simulink model "host_visualization"  (R2018b)
settings: Solver=FixedStepAuto  StartTime=0.0  StopTime=inf  FixedStep=0.002  RelTol=1e-3
model workspace (MAT data in the model file):
  P_Sim_LowPassVisualization = Simulink.Parameter
  P_Sim_LowPassVisualization.Value = 0.03
  P_Sim_LowPassVisualization.DataType = 'auto'
  P_Sim_LowPassVisualization.Dimensions = [1 1]
libraries: misc x6, sim3dlib x3, simulink x1, xpcrtudplib x1, xpcutilitieslib x1
settings Model: EnablePacing=on  Creator=speedgoat  LastModifiedBy=ge34qer

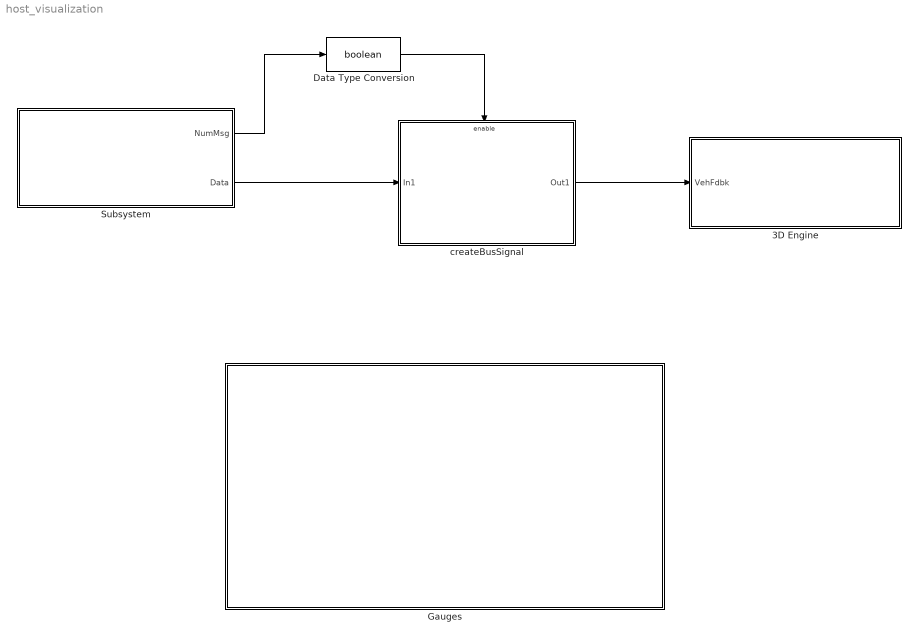
== system host_visualization ==
  3D Engine : Subsystem  VariantControlMode=Label  Variant=on  LabelModeActiveChoice=1  mask(3D Engine){engine3D=Enabled, SceneDesc=Straight road, dt3D=0.02}
      mask prompts: engine3D "3D Engine"; SceneDesc "Scene Description:"; dt3D "Engine frame rate, dt3D [s]:"
      mask help: This subsystem contains the interface blocks which permit the display of the vehicle in 3D virtual environment. Enable it to view the simulation progress, disable it to inhibit the display.
      mask init:
      | switch get_param(gcb,'engine3D')
      |     case 'Disabled'
      |         set_param(gcb,'OverrideUsingVariant','0')
      |         try
      |             set_param([bdroot '/Environment/Ground Feedback'],'OverrideUsingVariant','0')
      |         catch
      |             disp('No ground feedback sensor found')
      |         end
      |     case 'Enabled'
      |         set_param(gcb,'OverrideUsingVariant','1')
      |         try
      |             set_param([bdroot '/Environment/Ground Feedback'],'OverrideUsingVariant','1')
      |         catch
      |             disp('No ground feedback sensor found')
      |         end
      |     otherwise
      |         set_param(gcb,'OverrideUsingVariant','0')
      | end
      settings: AttributesFormatString=%<engine3D>
      mask Help: eval('vdynblkshelp(''vdynblksscenecameraray'')');
      mask TypeOptions engine3D: Enabled | Disabled
      mask Callback engine3D:
      | switch get_param(gcb,'engine3D')
      |     case 'Disabled'
      |         set_param(gcb,'OverrideUsingVariant','0')
      |     case 'Enabled'
      |        set_param(gcb,'OverrideUsingVariant','1')
      |     otherwise
      |        set_param(gcb,'OverrideUsingVariant','0')
      | end
      mask TypeOptions SceneDesc:
      | 3D Engine/Simulation 3D Engine
      | 1/SceneDesc
      mask Display: disp('3D Engine')
  Data Type Conversion : DataTypeConversion  OutDataTypeStr=boolean
  Gauges : Subsystem
  Subsystem : Subsystem
  createBusSignal : Subsystem
  wires:
  createBusSignal/1(Out1) -> 3D Engine/1(VehFdbk)
  Subsystem/1(NumMsg) -> Data Type Conversion/1
  Data Type Conversion/1 -> createBusSignal/Enable
  Subsystem/2(Data) -> createBusSignal/1(In1)

== system host_visualization/3D Engine ==
  note: 1) Add Subsystem or Model blocks as valid variant choices.
      | 2) You cannot connect blocks at this level. At simulation, connectivity is automatically
      | determined, based on the active variant and port name matching.
  VehFdbk : Inport
  3D Engine : Subsystem  VariantControl=1
  3D Engine Disabled : Subsystem  VariantControl=0

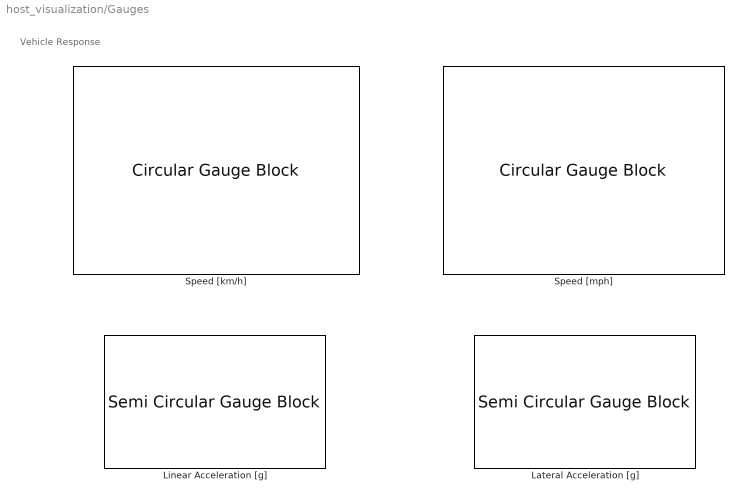
== system host_visualization/Gauges ==
  note: Vehicle Response
  Lateral Acceleration [g] : SemiCircularGaugeBlock  WebBlockId=331  LabelPosition=Hide  ScaleMin=-1.6000000000000001  ScaleMax=1.6000000000000001
  Linear Acceleration [g] : SemiCircularGaugeBlock  WebBlockId=343  LabelPosition=Hide  ScaleMin=-1.6000000000000001  ScaleMax=1.6000000000000001
  Speed [km/h] : CircularGaugeBlock  WebBlockId=332  LabelPosition=Hide  ScaleMax=210
  Speed [mph] : CircularGaugeBlock  WebBlockId=339  LabelPosition=Hide  ScaleMax=130

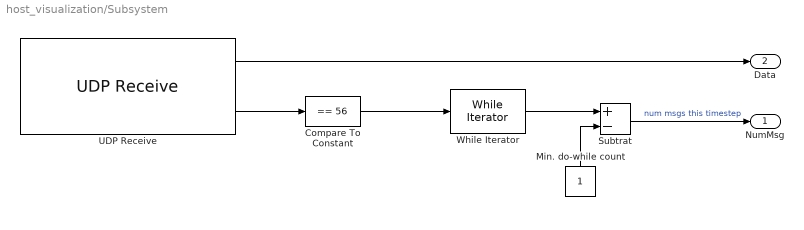
== system host_visualization/Subsystem ==
  Compare To Constant : simulink/Logic and Bit Operations/Compare To Constant  Priority=1  relop===  const=56  OutDataTypeStr=boolean
  Min. do-while count : Constant  OutDataTypeStr=int8  SampleTime=-1
  Subtrat : Sum  Inputs=+-
  UDP Receive : xpcrtudplib/UDP Receive  ipAddressVal=Use host-target connection  localPort=25000  rcvWidth=56  rcvFmAny=off  fmAddress=192.168.7.3  rcvMulticast=off  multicastAddress={}  maxUDPQueue=8  sampleTime=-1
      settings: SourceProductName=Simulink Real-Time
  While Iterator : WhileIterator  WhileBlockType=do-while  ShowIterationPort=on  OutputDataType=int16
  NumMsg : Outport
  Data : Outport  Port=2
  wires:
  Subtrat/1 -> NumMsg/1  "num msgs this timestep"
  Compare To Constant/1 -> While Iterator/1
  UDP Receive/1 -> Data/1
  Min. do-while count/1 -> Subtrat/2
  While Iterator/1 -> Subtrat/1
  UDP Receive/2 -> Compare To Constant/1

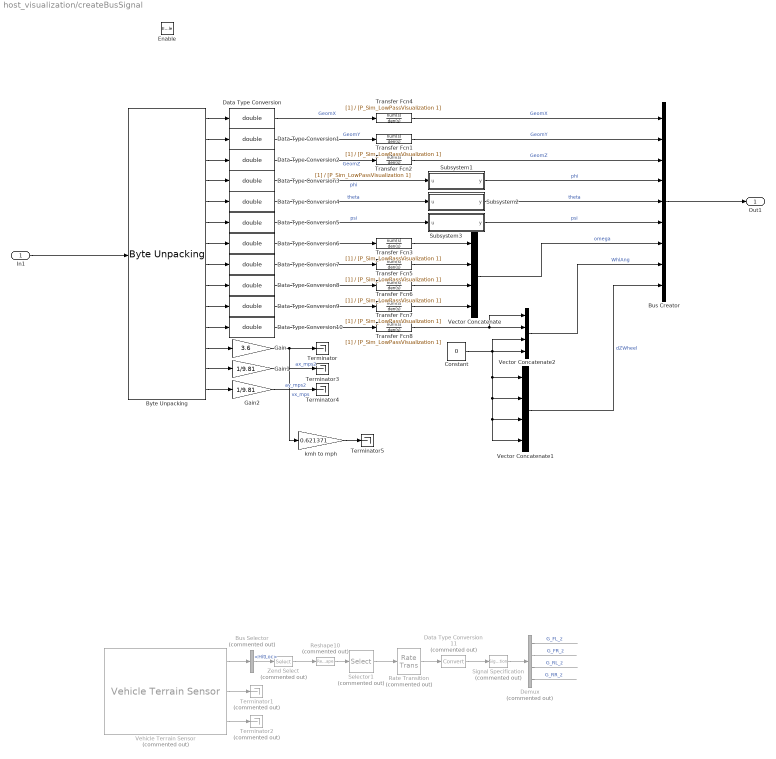
== system host_visualization/createBusSignal ==
  In1 : Inport
  Enable : EnablePort
  Bus Creator : BusCreator  Inputs=9
  Bus Selector : BusSelector  Commented=on  OutputSignals=HitLoc
  "Byte Unpacking " : xpcutilitieslib/Byte Unpacking   MaskUnpackedDataTypes={'single','single','single','single','single','single','single','single','single','single','single','single','single','single'}  MaskUnpackedDataSizes={[1],[1],[1],[1],[1],[1],[1],[1],[1],[1],[1],[1],[1],[1]}  MaskAlignment=1
      settings: SourceProductName=Simulink Real-Time  SourceProductBaseCode=XP
  Constant : Constant  Value=0  OutDataTypeStr=double  SampleTime=-1
  Data Type Conversion{,1..10} (11 alike) : DataTypeConversion  OutDataTypeStr=double
  Data Type Conversion11 : DataTypeConversion  Commented=on
  Demux : Demux  Commented=on
  Gain : Gain  Gain=3.6
  Gain1 : Gain  Gain=1/9.81
  Gain2 : Gain  Gain=1/9.81
  Rate Transition : RateTransition  Commented=on
  Reshape10 : Reshape  Commented=on  OutputDimensionality=Row vector (2-D)
  Selector1 : Selector  Commented=on  InputPortWidth=5  IndexOptions=Index vector (dialog)  Indices=[2:5]  OutputSizes=1
  Signal Specification : SignalSpecification  Commented=on  Unit=m
  Subsystem1 : Subsystem
  Subsystem2 : Subsystem
  Subsystem3 : Subsystem
  Terminator{,3..5} (4 alike) : Terminator
  Terminator1 : Terminator  Commented=on
  Terminator2 : Terminator  Commented=on
  Transfer Fcn{1..8} (8 alike) : TransferFcn  Denominator=[P_Sim_LowPassVisualization 1]
  Vector Concatenate : Concatenate  NumInputs=4
  Vector Concatenate1 : Concatenate  NumInputs=4
  Vector Concatenate2 : Concatenate  NumInputs=4
  Vehicle Terrain Sensor : sim3dlib/Vehicle Terrain Sensor  Commented=on  ActorTag=SimulinkVehicle1  VehExtEn=Constant  TireRadiiExt=Constant  VehCntrLngthVal=0  TireRadiiVal=0  VehRayLngth=10  LfRayLngth=20  RfRayLngth=20  LrRayLngth=20  RrRayLngth=20  VehRayOffset=0  LfRayOffset=-1  RfRayOffset=-1  LrRayOffset=-1  RrRayOffset=-1  VehEn=on  LfEn=on  RfEn=on  LrEn=on  RrEn=on  DbgEn=off  Ts=0.02
  Zend Select : Selector  Commented=on  NumberOfDimensions=2  InputPortWidth=3  IndexOptions=Select all,Index vector (dialog)  Indices=[1 3],3  OutputSizes=1,1
  kmh to mph : Gain  Gain=0.621371
  Out1 : Outport
  wires:
  In1/1 -> "Byte Unpacking "/1
  "Byte Unpacking "/1 -> Data Type Conversion/1
  "Byte Unpacking "/2 -> Data Type Conversion1/1
  "Byte Unpacking "/3 -> Data Type Conversion2/1
  "Byte Unpacking "/4 -> Data Type Conversion3/1
  "Byte Unpacking "/5 -> Data Type Conversion4/1
  "Byte Unpacking "/6 -> Data Type Conversion5/1
  "Byte Unpacking "/7 -> Data Type Conversion6/1
  "Byte Unpacking "/8 -> Data Type Conversion7/1
  "Byte Unpacking "/9 -> Data Type Conversion8/1
  "Byte Unpacking "/10 -> Data Type Conversion9/1
  Vector Concatenate/1 -> Bus Creator/7  "omega"
  Constant/1 -> Vector Concatenate1/1, Vector Concatenate1/2, Vector Concatenate1/3, Vector Concatenate1/4, Vector Concatenate2/4, Vector Concatenate2/3
  Vector Concatenate1/1 -> Bus Creator/9  "dZWheel"
  Bus Creator/1 -> Out1/1
  "Byte Unpacking "/11 -> Data Type Conversion10/1
  Vector Concatenate2/1 -> Bus Creator/8  "WhlAng"
  Data Type Conversion/1 -> Transfer Fcn4/1  "GeomX"
  Data Type Conversion1/1 -> Transfer Fcn1/1  "GeomY"
  Data Type Conversion2/1 -> Transfer Fcn2/1  "GeomZ"
  Data Type Conversion3/1 -> Subsystem1/1(u)  "phi"
  Data Type Conversion4/1 -> Subsystem2/1(u)  "theta"
  Data Type Conversion6/1 -> Transfer Fcn3/1
  Data Type Conversion7/1 -> Transfer Fcn5/1
  Data Type Conversion8/1 -> Transfer Fcn6/1
  Data Type Conversion9/1 -> Transfer Fcn7/1
  Data Type Conversion10/1 -> Transfer Fcn8/1
  Data Type Conversion5/1 -> Subsystem3/1(u)  "psi"
  Signal Specification/1 -> Demux/1
  Demux/3 -> ?  "G_RL_z"
  Vehicle Terrain Sensor/2 -> Terminator1/1
  Rate Transition/1 -> Data Type Conversion11/1
  Vehicle Terrain Sensor/3 -> Terminator2/1
  Bus Selector/1 -> Zend Select/1  "<HitLoc>"
  Reshape10/1 -> Selector1/1
  Demux/1 -> ?  "G_FL_z"
  Demux/2 -> ?  "G_FR_z"
  Zend Select/1 -> Reshape10/1
  Selector1/1 -> Rate Transition/1
  Data Type Conversion11/1 -> Signal Specification/1
  Vehicle Terrain Sensor/1 -> Bus Selector/1
  Demux/4 -> ?  "G_RR_z"
  Transfer Fcn4/1 -> Bus Creator/1  "GeomX"
  Transfer Fcn3/1 -> Vector Concatenate/1
  Transfer Fcn5/1 -> Vector Concatenate/2
  Transfer Fcn6/1 -> Vector Concatenate/3
  Transfer Fcn7/1 -> Vector Concatenate/4
  Transfer Fcn8/1 -> Vector Concatenate2/2, Vector Concatenate2/1
  Transfer Fcn1/1 -> Bus Creator/2  "GeomY"
  Transfer Fcn2/1 -> Bus Creator/3  "GeomZ"
  Subsystem1/1(y) -> Bus Creator/4  "phi"
  Subsystem2/1(y) -> Bus Creator/5  "theta"
  Subsystem3/1(y) -> Bus Creator/6  "psi"
  Gain/1 -> kmh to mph/1, Terminator/1  "vx_mps"
  "Byte Unpacking "/13 -> Gain1/1
  "Byte Unpacking "/14 -> Gain2/1
  "Byte Unpacking "/12 -> Gain/1
  Gain1/1 -> Terminator3/1  "ax_mps2"
  Gain2/1 -> Terminator4/1  "ay_mps2"
  kmh to mph/1 -> Terminator5/1

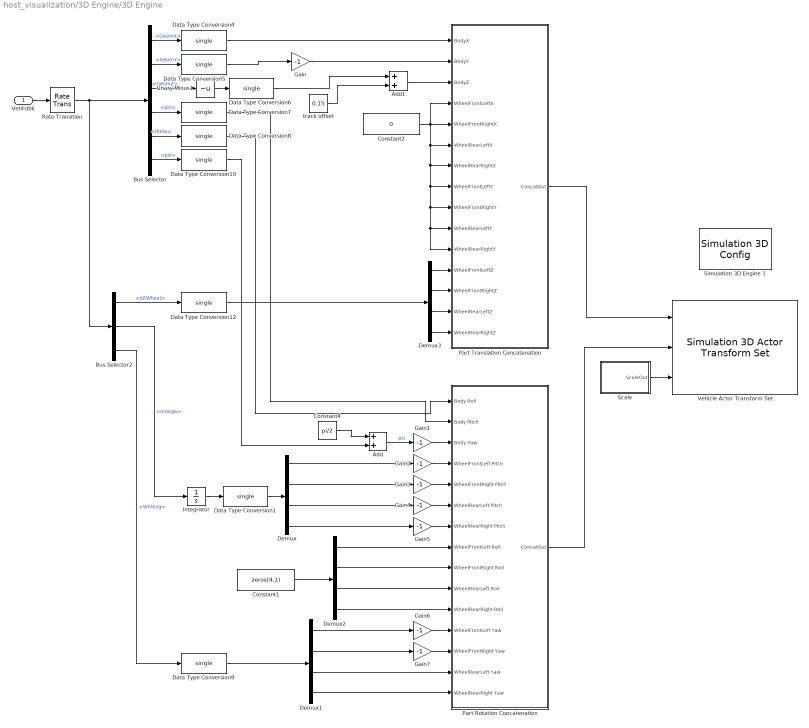
== system host_visualization/3D Engine/3D Engine ==
  VehFdbk : Inport
  Add : Sum
  Add1 : Sum
  Bus Selector : BusSelector  OutputSignals=GeomX,GeomY,GeomZ,phi,theta,psi
  Bus Selector2 : BusSelector  OutputSignals=dZWheel,omega,WhlAng
  Constant1 : Constant  Value=zeros(4,1)  OutDataTypeStr=single
  Constant2 : Constant  Value=0  OutDataTypeStr=single
  Constant4 : Constant  Value=pi/2  OutDataTypeStr=single
  Data Type Conversion{1,4..10,12} (9 alike) : DataTypeConversion  OutDataTypeStr=single
  Demux{,1..3} (4 alike) : Demux
  Gain{,1..7} (8 alike) : Gain  Gain=-1
  Integrator : Integrator  WrapState=on  WrappedStateUpperValue=2*pi  WrappedStateLowerValue=0  ZeroCross=off
  Part Rotation Concatenation : Subsystem
  Part Translation Concatenation : Subsystem
  Rate Transition : RateTransition  OutPortSampleTime=dt3D
  Scale : Subsystem
  Simulation 3D Engine 1 : sim3dlib/Simulation 3D Config  Priority=1  ProjectFormat=Executable  ProjectName=C:\Users\speedgoat\Desktop\testbuild2\WindowsNoEditor\AutoVrtlEnv.exe /Game/Maps/fancy_monteblanco  SceneDesc=Straight road  OpVisEn=off  Ts=dt3D
      settings: AttributesFormatString=Priority: %<Priority>
  Unary Minus1 : UnaryMinus
  Vehicle Actor Transform Set : sim3dlib/Simulation 3D Actor Transform Set  ActorTag=SimulinkVehicle1  ActorType=Passenger vehicle  PassVehMesh=Muscle car  VehColor=Silver  NumberOfParts=5  CustNumOfParts=3  Translation=[0 0 1; 0 0 0; 0 0 0; 0 0 0; 0 0 0]  Rotation=[0 0 0; 0 0 0; 0 0 0; 0 0 0; 0 0 0]  Scale=[1 1 1; 1 1 1; 1 1 1; 1 1 1; 1 1 1]  Ts=dt3D
  track offset : Constant  Value=0.15  OutDataTypeStr=single
  wires:
  Bus Selector/5 -> Data Type Conversion8/1  "<theta>"
  Bus Selector/6 -> Data Type Conversion10/1  "<psi>"
  Bus Selector/3 -> Unary Minus1/1  "<GeomZ>"
  Bus Selector/2 -> Data Type Conversion5/1  "<GeomY>"
  Bus Selector/1 -> Data Type Conversion4/1  "<GeomX>"
  Data Type Conversion7/1 -> Part Rotation Concatenation/2(Body Ptich)
  Constant2/1 -> Part Translation Concatenation/4(WheelFrontLeftX), Part Translation Concatenation/6(WheelRearLeftX), Part Translation Concatenation/7(WheelRearRightX), Part Translation Concatenation/8(WheelFrontLeftY), Part Translation Concatenation/9(WheelFrontRightY), Part Translation Concatenation/10(WheelRearLeftY), Part Translation Concatenation/11(WheelRearRightY), Part Translation Concatenation/5(WheelFrontRightX)
  Data Type Conversion10/1 -> Add/2
  Data Type Conversion8/1 -> Part Rotation Concatenation/1(Body Roll)
  Data Type Conversion1/1 -> Demux/1
  Integrator/1 -> Data Type Conversion1/1
  Demux1/2 -> Gain7/1
  Demux1/1 -> Gain6/1
  Data Type Conversion9/1 -> Demux1/1
  Bus Selector2/2 -> Integrator/1  "<omega>"
  Bus Selector2/3 -> Data Type Conversion9/1  "<WhlAng>"
  Demux2/4 -> Part Rotation Concatenation/11(WheelRearRight Roll)
  Demux2/3 -> Part Rotation Concatenation/10(WheelRearLeft Roll)
  Demux2/2 -> Part Rotation Concatenation/9(WheelFrontRight Roll)
  Demux2/1 -> Part Rotation Concatenation/8(WheelFrontLeft Roll)
  Demux1/3 -> Part Rotation Concatenation/14(WheelRearLeft Yaw)
  Demux1/4 -> Part Rotation Concatenation/15(WheelRearRight Yaw)
  VehFdbk/1 -> Rate Transition/1
  Demux3/2 -> Part Translation Concatenation/13(WheelFrontRightZ)
  Demux3/1 -> Part Translation Concatenation/12(WheelFrontLeftZ)
  Demux3/3 -> Part Translation Concatenation/14(WheelRearLeftZ)
  Demux3/4 -> Part Translation Concatenation/15(WheelRearRightZ)
  Data Type Conversion12/1 -> Demux3/1
  Part Translation Concatenation/1(ConcatOut) -> Vehicle Actor Transform Set/1
  Part Rotation Concatenation/1(ConcatOut) -> Vehicle Actor Transform Set/2
  Bus Selector/4 -> Data Type Conversion7/1  "<phi>"
  Constant1/1 -> Demux2/1
  Demux/1 -> Gain2/1
  Demux/2 -> Gain3/1
  Demux/3 -> Gain4/1
  Demux/4 -> Gain5/1
  Scale/1(ScaleOut) -> Vehicle Actor Transform Set/3
  Rate Transition/1 -> Bus Selector2/1, Bus Selector/1
  Bus Selector2/1 -> Data Type Conversion12/1  "<dZWheel>"
  Unary Minus1/1 -> Data Type Conversion6/1
  Data Type Conversion4/1 -> Part Translation Concatenation/1(BodyX)
  Data Type Conversion5/1 -> Gain/1
  Gain/1 -> Part Translation Concatenation/2(BodyY)
  Constant4/1 -> Add/1
  Add/1 -> Gain1/1  "psi"
  Gain1/1 -> Part Rotation Concatenation/3(Body Yaw)
  Gain2/1 -> Part Rotation Concatenation/4(WheelFrontLeft Pitch)
  Gain3/1 -> Part Rotation Concatenation/5(WheelFrontRight Pitch)
  Gain4/1 -> Part Rotation Concatenation/6(WheelRearLeft Pitch)
  Gain5/1 -> Part Rotation Concatenation/7(WheelRearRight Ptich)
  Gain6/1 -> Part Rotation Concatenation/12(WheelFrontLeft Yaw)
  Gain7/1 -> Part Rotation Concatenation/13(WheelFrontRight Yaw)
  track offset/1 -> Add1/2
  Data Type Conversion6/1 -> Add1/1
  Add1/1 -> Part Translation Concatenation/3(BodyZ)

== system host_visualization/3D Engine/3D Engine Disabled ==
  VehFdbk : Inport
  Terminator : Terminator
  wires:
  VehFdbk/1 -> Terminator/1

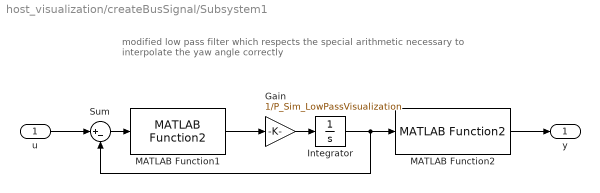
== system host_visualization/createBusSignal/Subsystem1 ==
  note: modified low pass filter which respects the special arithmetic necessary
      | to interpolate the yaw angle correctly
  u : Inport
  Gain : Gain  Gain=1/P_Sim_LowPassVisualization
  Integrator : Integrator
  MATLAB Function1 : misc/MATLAB Function2  SystemSampleTime=-1
  MATLAB Function2 : misc/MATLAB Function2  SystemSampleTime=-1
  Sum : Sum  Inputs=|+-
  y : Outport
  wires:
  Sum/1 -> MATLAB Function1/1
  MATLAB Function1/1 -> Gain/1
  Integrator/1 -> MATLAB Function2/1, Sum/2
  Gain/1 -> Integrator/1
  MATLAB Function2/1 -> y/1
  u/1 -> Sum/1

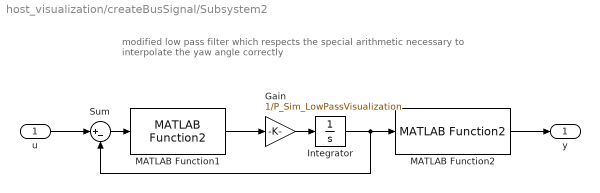
== system host_visualization/createBusSignal/Subsystem2 ==
  note: modified low pass filter which respects the special arithmetic necessary
      | to interpolate the yaw angle correctly
  u : Inport
  Gain : Gain  Gain=1/P_Sim_LowPassVisualization
  Integrator : Integrator
  MATLAB Function1 : misc/MATLAB Function2  SystemSampleTime=-1
  MATLAB Function2 : misc/MATLAB Function2  SystemSampleTime=-1
  Sum : Sum  Inputs=|+-
  y : Outport
  wires:
  Sum/1 -> MATLAB Function1/1
  MATLAB Function1/1 -> Gain/1
  Integrator/1 -> MATLAB Function2/1, Sum/2
  Gain/1 -> Integrator/1
  MATLAB Function2/1 -> y/1
  u/1 -> Sum/1

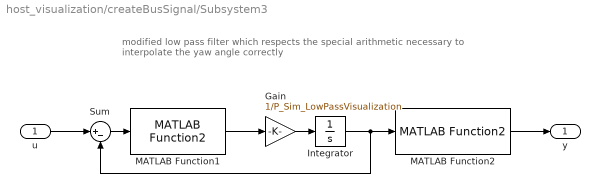
== system host_visualization/createBusSignal/Subsystem3 ==
  note: modified low pass filter which respects the special arithmetic necessary
      | to interpolate the yaw angle correctly
  u : Inport
  Gain : Gain  Gain=1/P_Sim_LowPassVisualization
  Integrator : Integrator
  MATLAB Function1 : misc/MATLAB Function2  SystemSampleTime=-1
  MATLAB Function2 : misc/MATLAB Function2  SystemSampleTime=-1
  Sum : Sum  Inputs=|+-
  y : Outport
  wires:
  Sum/1 -> MATLAB Function1/1
  MATLAB Function1/1 -> Gain/1
  Integrator/1 -> MATLAB Function2/1, Sum/2
  Gain/1 -> Integrator/1
  MATLAB Function2/1 -> y/1
  u/1 -> Sum/1

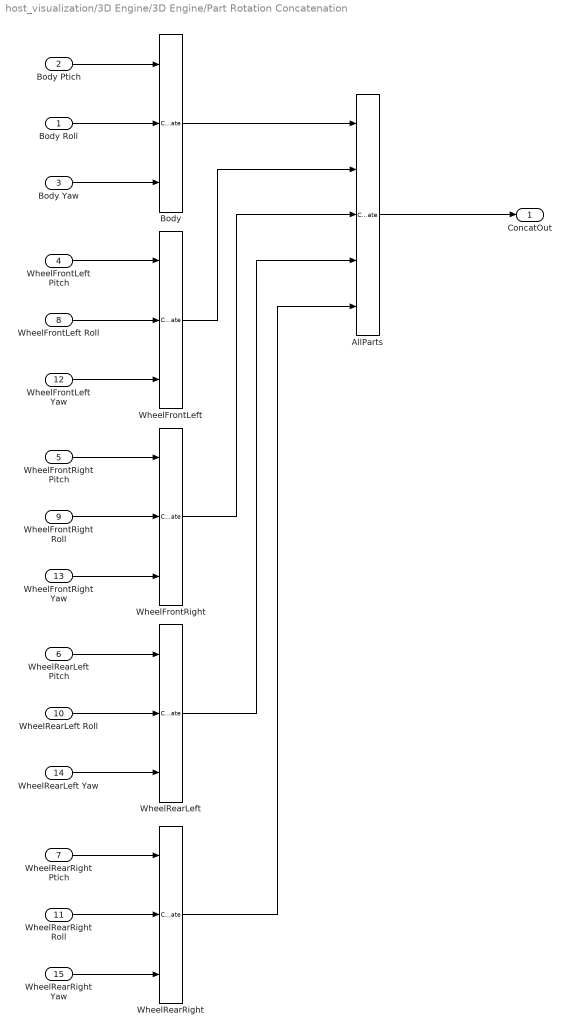
== system host_visualization/3D Engine/3D Engine/Part Rotation Concatenation ==
  Body Roll : Inport
  Body Ptich : Inport  Port=2
  Body Yaw : Inport  Port=3
  WheelFrontLeft Pitch : Inport  Port=4
  WheelFrontRight Pitch : Inport  Port=5
  WheelRearLeft Pitch : Inport  Port=6
  WheelRearRight Ptich : Inport  Port=7
  WheelFrontLeft Roll : Inport  Port=8
  WheelFrontRight Roll : Inport  Port=9
  WheelRearLeft Roll : Inport  Port=10
  WheelRearRight Roll : Inport  Port=11
  WheelFrontLeft Yaw : Inport  Port=12
  WheelFrontRight Yaw : Inport  Port=13
  WheelRearLeft Yaw : Inport  Port=14
  WheelRearRight Yaw : Inport  Port=15
  AllParts : Concatenate  NumInputs=5  Mode=Multidimensional array
  Body : Concatenate  NumInputs=3  Mode=Multidimensional array  ConcatenateDimension=2
  WheelFrontLeft : Concatenate  NumInputs=3  Mode=Multidimensional array  ConcatenateDimension=2
  WheelFrontRight : Concatenate  NumInputs=3  Mode=Multidimensional array  ConcatenateDimension=2
  WheelRearLeft : Concatenate  NumInputs=3  Mode=Multidimensional array  ConcatenateDimension=2
  WheelRearRight : Concatenate  NumInputs=3  Mode=Multidimensional array  ConcatenateDimension=2
  ConcatOut : Outport
  wires:
  WheelFrontRight Yaw/1 -> WheelFrontRight/3
  WheelRearLeft Pitch/1 -> WheelRearLeft/1
  WheelRearRight/1 -> AllParts/5
  WheelRearLeft Roll/1 -> WheelRearLeft/2
  AllParts/1 -> ConcatOut/1
  WheelRearLeft Yaw/1 -> WheelRearLeft/3
  WheelRearRight Roll/1 -> WheelRearRight/2
  WheelFrontRight Pitch/1 -> WheelFrontRight/1
  WheelFrontRight Roll/1 -> WheelFrontRight/2
  WheelRearRight Yaw/1 -> WheelRearRight/3
  WheelFrontRight/1 -> AllParts/3
  WheelRearLeft/1 -> AllParts/4
  Body/1 -> AllParts/1
  WheelRearRight Ptich/1 -> WheelRearRight/1
  WheelFrontLeft/1 -> AllParts/2
  Body Roll/1 -> Body/2
  WheelFrontLeft Roll/1 -> WheelFrontLeft/2
  WheelFrontLeft Yaw/1 -> WheelFrontLeft/3
  WheelFrontLeft Pitch/1 -> WheelFrontLeft/1
  Body Yaw/1 -> Body/3
  Body Ptich/1 -> Body/1

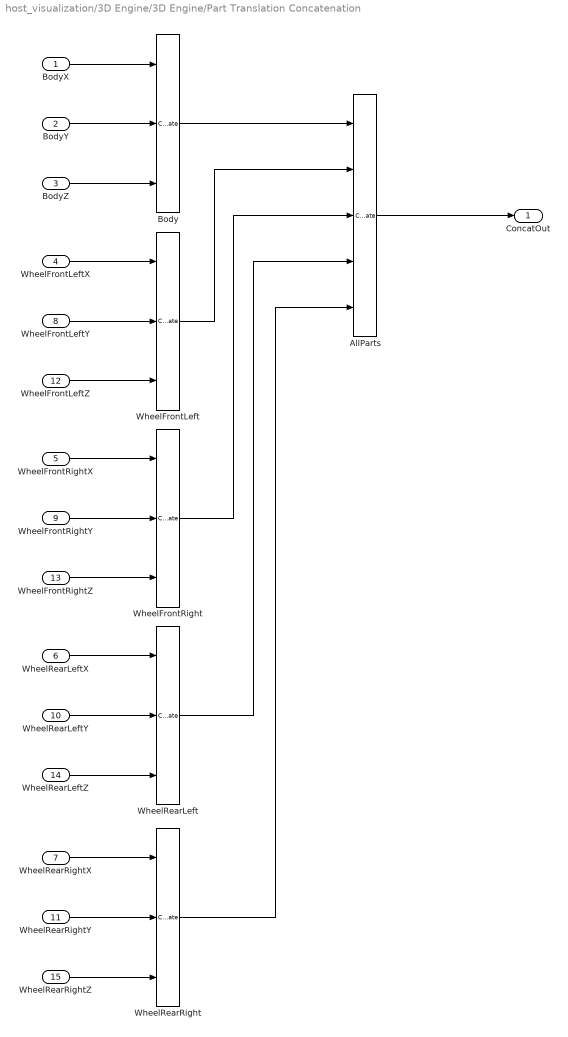
== system host_visualization/3D Engine/3D Engine/Part Translation Concatenation ==
  BodyX : Inport
  BodyY : Inport  Port=2
  BodyZ : Inport  Port=3
  WheelFrontLeftX : Inport  Port=4
  WheelFrontRightX : Inport  Port=5
  WheelRearLeftX : Inport  Port=6
  WheelRearRightX : Inport  Port=7
  WheelFrontLeftY : Inport  Port=8
  WheelFrontRightY : Inport  Port=9
  WheelRearLeftY : Inport  Port=10
  WheelRearRightY : Inport  Port=11
  WheelFrontLeftZ : Inport  Port=12
  WheelFrontRightZ : Inport  Port=13
  WheelRearLeftZ : Inport  Port=14
  WheelRearRightZ : Inport  Port=15
  AllParts : Concatenate  NumInputs=5  Mode=Multidimensional array
  Body : Concatenate  NumInputs=3  Mode=Multidimensional array  ConcatenateDimension=2
  WheelFrontLeft : Concatenate  NumInputs=3  Mode=Multidimensional array  ConcatenateDimension=2
  WheelFrontRight : Concatenate  NumInputs=3  Mode=Multidimensional array  ConcatenateDimension=2
  WheelRearLeft : Concatenate  NumInputs=3  Mode=Multidimensional array  ConcatenateDimension=2
  WheelRearRight : Concatenate  NumInputs=3  Mode=Multidimensional array  ConcatenateDimension=2
  ConcatOut : Outport
  wires:
  WheelFrontRightZ/1 -> WheelFrontRight/3
  WheelRearLeftX/1 -> WheelRearLeft/1
  WheelRearRight/1 -> AllParts/5
  WheelRearLeftY/1 -> WheelRearLeft/2
  AllParts/1 -> ConcatOut/1
  WheelRearLeftZ/1 -> WheelRearLeft/3
  WheelRearRightY/1 -> WheelRearRight/2
  WheelFrontRightX/1 -> WheelFrontRight/1
  WheelFrontRightY/1 -> WheelFrontRight/2
  WheelRearRightZ/1 -> WheelRearRight/3
  WheelFrontRight/1 -> AllParts/3
  WheelRearLeft/1 -> AllParts/4
  Body/1 -> AllParts/1
  WheelRearRightX/1 -> WheelRearRight/1
  WheelFrontLeft/1 -> AllParts/2
  BodyY/1 -> Body/2
  WheelFrontLeftY/1 -> WheelFrontLeft/2
  WheelFrontLeftZ/1 -> WheelFrontLeft/3
  WheelFrontLeftX/1 -> WheelFrontLeft/1
  BodyZ/1 -> Body/3
  BodyX/1 -> Body/1

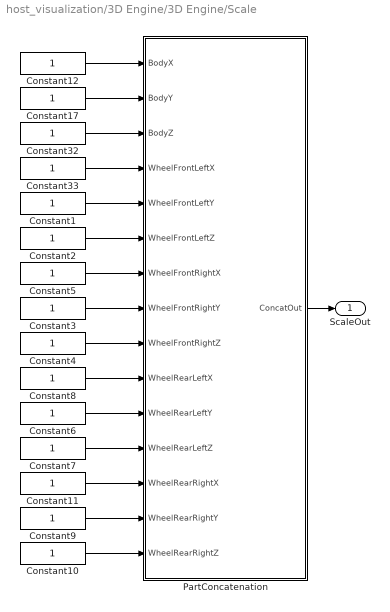
== system host_visualization/3D Engine/3D Engine/Scale ==
  Constant{1..12,17,32..33} (15 alike) : Constant  OutDataTypeStr=single
  PartConcatenation : Subsystem
  ScaleOut : Outport
  wires:
  PartConcatenation/1(ConcatOut) -> ScaleOut/1
  Constant12/1 -> PartConcatenation/1(BodyX)
  Constant17/1 -> PartConcatenation/2(BodyY)
  Constant32/1 -> PartConcatenation/3(BodyZ)
  Constant33/1 -> PartConcatenation/4(WheelFrontLeftX)
  Constant1/1 -> PartConcatenation/5(WheelFrontLeftY)
  Constant2/1 -> PartConcatenation/6(WheelFrontLeftZ)
  Constant5/1 -> PartConcatenation/7(WheelFrontRightX)
  Constant3/1 -> PartConcatenation/8(WheelFrontRightY)
  Constant4/1 -> PartConcatenation/9(WheelFrontRightZ)
  Constant8/1 -> PartConcatenation/10(WheelRearLeftX)
  Constant6/1 -> PartConcatenation/11(WheelRearLeftY)
  Constant7/1 -> PartConcatenation/12(WheelRearLeftZ)
  Constant11/1 -> PartConcatenation/13(WheelRearRightX)
  Constant9/1 -> PartConcatenation/14(WheelRearRightY)
  Constant10/1 -> PartConcatenation/15(WheelRearRightZ)

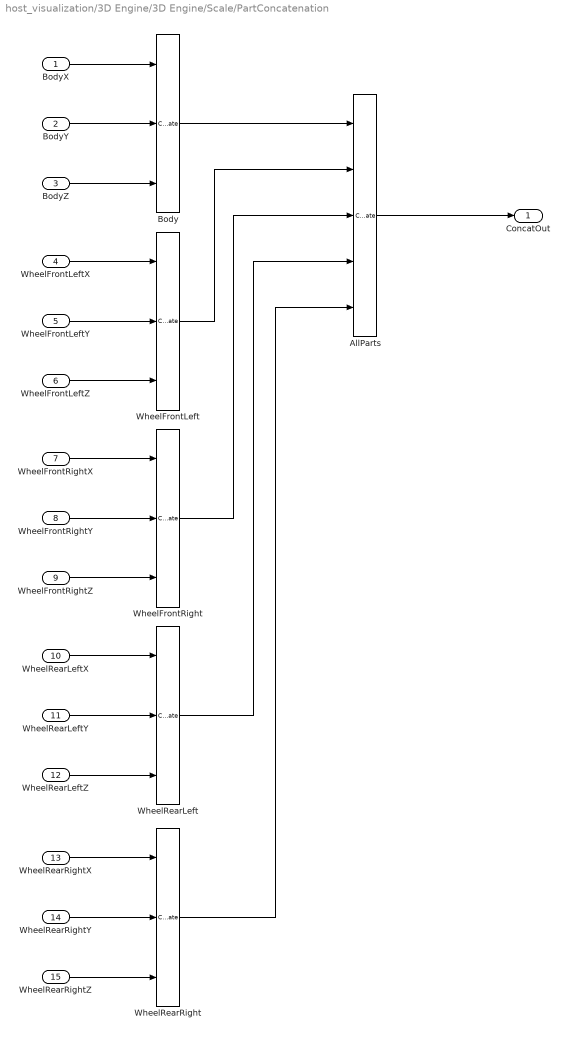
== system host_visualization/3D Engine/3D Engine/Scale/PartConcatenation ==
  BodyX : Inport
  BodyY : Inport  Port=2
  BodyZ : Inport  Port=3
  WheelFrontLeftX : Inport  Port=4
  WheelFrontLeftY : Inport  Port=5
  WheelFrontLeftZ : Inport  Port=6
  WheelFrontRightX : Inport  Port=7
  WheelFrontRightY : Inport  Port=8
  WheelFrontRightZ : Inport  Port=9
  WheelRearLeftX : Inport  Port=10
  WheelRearLeftY : Inport  Port=11
  WheelRearLeftZ : Inport  Port=12
  WheelRearRightX : Inport  Port=13
  WheelRearRightY : Inport  Port=14
  WheelRearRightZ : Inport  Port=15
  AllParts : Concatenate  NumInputs=5  Mode=Multidimensional array
  Body : Concatenate  NumInputs=3  Mode=Multidimensional array  ConcatenateDimension=2
  WheelFrontLeft : Concatenate  NumInputs=3  Mode=Multidimensional array  ConcatenateDimension=2
  WheelFrontRight : Concatenate  NumInputs=3  Mode=Multidimensional array  ConcatenateDimension=2
  WheelRearLeft : Concatenate  NumInputs=3  Mode=Multidimensional array  ConcatenateDimension=2
  WheelRearRight : Concatenate  NumInputs=3  Mode=Multidimensional array  ConcatenateDimension=2
  ConcatOut : Outport
  wires:
  WheelFrontRightZ/1 -> WheelFrontRight/3
  WheelRearLeftX/1 -> WheelRearLeft/1
  WheelRearRight/1 -> AllParts/5
  WheelRearLeftY/1 -> WheelRearLeft/2
  AllParts/1 -> ConcatOut/1
  WheelRearLeftZ/1 -> WheelRearLeft/3
  WheelRearRightY/1 -> WheelRearRight/2
  WheelFrontRightX/1 -> WheelFrontRight/1
  WheelFrontRightY/1 -> WheelFrontRight/2
  WheelRearRightZ/1 -> WheelRearRight/3
  WheelFrontRight/1 -> AllParts/3
  WheelRearLeft/1 -> AllParts/4
  Body/1 -> AllParts/1
  WheelRearRightX/1 -> WheelRearRight/1
  WheelFrontLeft/1 -> AllParts/2
  BodyY/1 -> Body/2
  WheelFrontLeftY/1 -> WheelFrontLeft/2
  WheelFrontLeftZ/1 -> WheelFrontLeft/3
  WheelFrontLeftX/1 -> WheelFrontLeft/1
  BodyZ/1 -> Body/3
  BodyX/1 -> Body/1
